simulink model "hw"  (R2021a)
settings: Solver=VariableStepAuto  StartTime=0.0  StopTime=50  RelTol=1e-3
libraries: cstblocks x1
settings Model: Creator=HASEE  LastModifiedBy=HASEE

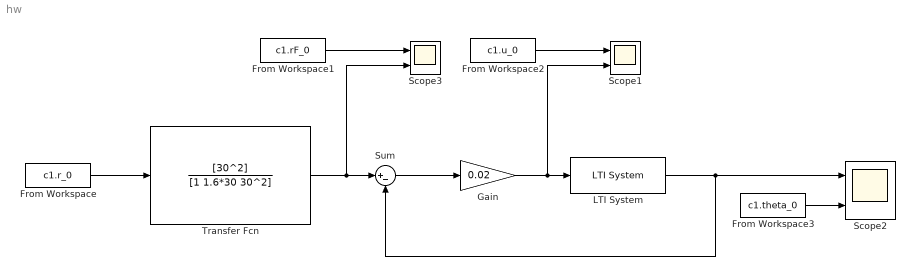
== system hw ==
  From Workspace : FromWorkspace  VariableName=c1.r_0
  From Workspace1 : FromWorkspace  VariableName=c1.rF_0
  From Workspace2 : FromWorkspace  VariableName=c1.u_0
  From Workspace3 : FromWorkspace  VariableName=c1.theta_0
  Gain : Gain  Gain=0.02
  LTI System : cstblocks/LTI System  sys=P1  IC=[]
  Scope1 : Scope  NumInputPorts=2
  Scope2 : Scope  NumInputPorts=2
  Scope3 : Scope  NumInputPorts=2
  Sum : Sum  Inputs=|+-
  Transfer Fcn : TransferFcn  Numerator=[30^2]  Denominator=[1 1.6*30 30^2]
  wires:
  From Workspace/1 -> Transfer Fcn/1
  Transfer Fcn/1 -> Scope3/2, Sum/1
  From Workspace1/1 -> Scope3/1
  Sum/1 -> Gain/1
  LTI System/1 -> Sum/2, Scope2/1
  From Workspace2/1 -> Scope1/1
  Gain/1 -> Scope1/2, LTI System/1
  From Workspace3/1 -> Scope2/2
